simulink library "csu_tpl_thruster_propellant_lander_lib"  (R2014b)
settings: Solver=ode45  StartTime=0.0  StopTime=10.0  RelTol=1e-3
values from neighbouring files (symbols this model uses):
  tpl_coarse_acs_thrust_to_isp = [ ... (first row only)    [csu_tpl_thruster_propellant_lander_prep.m]
  tpl_main_biprop_thrust_to_isp = [ 0           tpl_main_biprop_isp ... (first row only)    [csu_tpl_thruster_propellant_lander_prep.m]
  tpl_main_monoprop_thrust_to_isp = [ 0           tpl_main_monoprop_isp ... (first row only)    [csu_tpl_thruster_propellant_lander_prep.m]
  tpl_rp1_to_htp_ratio = 1/7.5    (= 0.133333333333)    [csu_tpl_thruster_propellant_lander_init.m]
  tpl_vernier_acs_thrust_to_isp = [ ... (first row only)    [csu_tpl_thruster_propellant_lander_prep.m]
libraries: util_info_lib x1
settings Model: Creator=Mark Agbayani  LastModifiedBy=jimkaidy

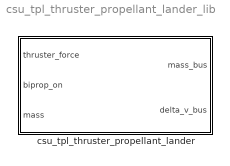
== system csu_tpl_thruster_propellant_lander_lib ==
  csu_tpl_thruster_propellant_lander : Subsystem

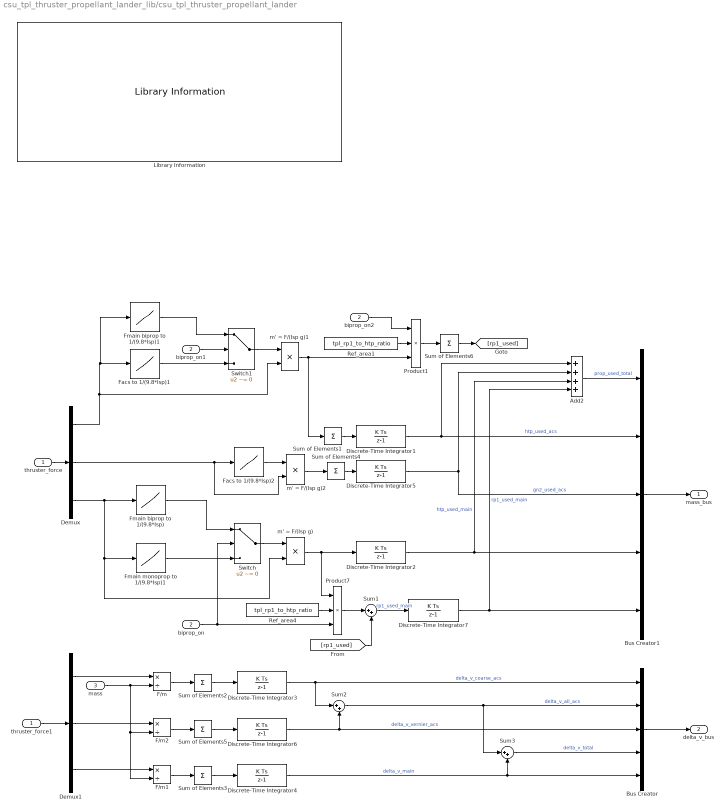
== system csu_tpl_thruster_propellant_lander_lib/csu_tpl_thruster_propellant_lander ==
  thruster_force : Inport
  biprop_on : Inport  Port=2
  mass : Inport  Port=3
  Add2 : Sum  Inputs=++++
  Bus Creator : BusCreator  Inputs=5
  Bus Creator1 : BusCreator  Inputs=5
  Demux : Demux  Outputs=[12 12 1]
  Demux1 : Demux  Outputs=[12 12 1]
  Discrete-Time Integrator{1..7} (7 alike) : DiscreteIntegrator  gainval=1  SampleTime=-1
  F/m : Product  Inputs=*/
  F/m1 : Product  Inputs=*/
  F/m2 : Product  Inputs=*/
  Facs to 1/(9.8*Isp)1 : Lookup  InputValues=tpl_coarse_acs_thrust_to_isp(:,1)  Table=1./(9.8*tpl_coarse_acs_thrust_to_isp(:,2))  LookUpMeth=Interpolation-Use End Values
  Facs to 1/(9.8*Isp)2 : Lookup  InputValues=tpl_vernier_acs_thrust_to_isp(:,1)  Table=1./(9.8*tpl_vernier_acs_thrust_to_isp(:,2))  LookUpMeth=Interpolation-Use End Values
  Fmain biprop to 1/(9.8*Isp) : Lookup  InputValues=tpl_main_biprop_thrust_to_isp(:,1)  Table=1./(9.8*tpl_main_biprop_thrust_to_isp(:,2))  LookUpMeth=Interpolation-Use End Values
  Fmain biprop to 1/(9.8*Isp)1 : Lookup  InputValues=tpl_main_biprop_thrust_to_isp(:,1)  Table=1./(9.8*tpl_main_biprop_thrust_to_isp(:,2))  LookUpMeth=Interpolation-Use End Values
  Fmain monoprop to 1/(9.8*Isp)1 : Lookup  InputValues=tpl_main_monoprop_thrust_to_isp(:,1)  Table=1./(9.8*tpl_main_monoprop_thrust_to_isp(:,2))  LookUpMeth=Interpolation-Use End Values
  Library Information : util_info_lib/Library Information  owner='NONE'
  Product1 : Product  Inputs=3  RndMeth=Zero
  Product7 : Product  Inputs=3  RndMeth=Zero
  Ref_area1 : Constant  Value=tpl_rp1_to_htp_ratio
  Ref_area4 : Constant  Value=tpl_rp1_to_htp_ratio
  Sum of Elements{1..6} (6 alike) : Sum  Inputs=+
  Sum1 : Sum  Inputs=|++
  Sum2 : Sum  Inputs=|++
  Sum3 : Sum  Inputs=|++
  Switch : Switch  Criteria=u2 ~= 0
  Switch1 : Switch  Criteria=u2 ~= 0
  biprop_on1 : InportShadow  Port=2
  biprop_on2 : InportShadow  Port=2
  m' = F/(Isp g) : Product  RndMeth=Zero
  m' = F/(Isp g)1 : Product  RndMeth=Zero
  m' = F/(Isp g)2 : Product  RndMeth=Zero
  thruster_force1 : InportShadow
  mass_bus : Outport
  delta_v_bus : Outport  Port=2
  wires:
  biprop_on/1 -> Switch/2, Product7/3
  Discrete-Time Integrator5/1 -> Add2/2, Bus Creator1/3  "gn2_used_acs"
  Sum1/1 -> Discrete-Time Integrator7/1  "rp1_used_main"
  Ref_area4/1 -> Product7/2
  Product7/1 -> Sum1/1
  Bus Creator1/1 -> mass_bus/1
  Bus Creator/1 -> delta_v_bus/1
  m' = F/(Isp g)2/1 -> Sum of Elements4/1
  Discrete-Time Integrator4/1 -> Bus Creator/5, Sum3/2  "delta_v_main"
  Demux1/3 -> F/m1/1
  Sum of Elements3/1 -> Discrete-Time Integrator4/1
  F/m1/1 -> Sum of Elements3/1
  Sum3/1 -> Bus Creator/4  "delta_v_total"
  Sum of Elements2/1 -> Discrete-Time Integrator3/1
  F/m/1 -> Sum of Elements2/1
  Demux1/1 -> F/m/1
  thruster_force1/1 -> Demux1/1
  mass/1 -> F/m2/2, F/m1/2, F/m/2
  Discrete-Time Integrator2/1 -> Bus Creator1/4, Add2/3  "htp_used_main"
  Sum of Elements1/1 -> Discrete-Time Integrator1/1
  Demux/1 -> Fmain biprop to 1/(9.8*Isp)1/1, Facs to 1/(9.8*Isp)1/1, m' = F/(Isp g)1/2
  m' = F/(Isp g)/1 -> Product7/1, Discrete-Time Integrator2/1
  thruster_force/1 -> Demux/1
  Add2/1 -> Bus Creator1/1  "prop_used_total"
  Demux/3 -> Fmain biprop to 1/(9.8*Isp)/1, Fmain monoprop to 1/(9.8*Isp)1/1, m' = F/(Isp g)/2
  Switch/1 -> m' = F/(Isp g)/1
  Fmain biprop to 1/(9.8*Isp)/1 -> Switch/1
  Fmain monoprop to 1/(9.8*Isp)1/1 -> Switch/3
  Sum of Elements4/1 -> Discrete-Time Integrator5/1
  Demux/2 -> Facs to 1/(9.8*Isp)2/1, m' = F/(Isp g)2/2
  Facs to 1/(9.8*Isp)2/1 -> m' = F/(Isp g)2/1
  Discrete-Time Integrator1/1 -> Add2/1, Bus Creator1/2  "htp_used_acs"
  Sum of Elements5/1 -> Discrete-Time Integrator6/1
  F/m2/1 -> Sum of Elements5/1
  Demux1/2 -> F/m2/1
  Discrete-Time Integrator6/1 -> Bus Creator/3, Sum2/2  "delta_v_vernier_acs"
  Discrete-Time Integrator3/1 -> Bus Creator/1, Sum2/1  "delta_v_coarse_acs"
  Sum2/1 -> Bus Creator/2, Sum3/1  "delta_v_all_acs"
  Switch1/1 -> m' = F/(Isp g)1/1
  biprop_on1/1 -> Switch1/2
  Facs to 1/(9.8*Isp)1/1 -> Switch1/3
  Fmain biprop to 1/(9.8*Isp)1/1 -> Switch1/1
  Ref_area1/1 -> Product1/2
  biprop_on2/1 -> Product1/1
  m' = F/(Isp g)1/1 -> Sum of Elements1/1, Product1/3
  Product1/1 -> Sum of Elements6/1
  [rp1_used] -> Sum1/2
  Sum of Elements6/1 -> [rp1_used]
  Discrete-Time Integrator7/1 -> Add2/4, Bus Creator1/5  "rp1_used_main"
